simulink model "sparam_filter_rab"  (Simulink 7.4)
settings: Solver=ode45  StartTime=0.0  StopTime=10  RelTol=1e-3
undefined symbols (not defined in the file or in its folder): Fs, magnitude, read, rfdata
libraries: dspindex x6, dspsigops x3, dspsnks4 x2, rfports1 x2, dspbuff3 x2, dspxfrm3 x2, dsparch3 x2, rfblackbox1 x1, simulink x1, dspmtrx3 x1, dspsrcs4 x1
settings Model: Creator=mikem  LastModifiedBy=Dick
settings DataIOCC: SaveOutput=off  SaveTime=off  SignalLoggingName=sigsOut
settings OptimizationCC: InlineInvariantSignals=on  InitFltsAndDblsToZero=on
settings DebuggingCC: SaveWithParameterizedLinksMsg=none  CheckExecutionContextPreStartOutputMsg=on  CheckExecutionContextRuntimeOutputMsg=on  SignalResolutionControl=TryResolveAllWithWarning  SolverPrmCheckMsg=none  MultiTaskDSMMsg=warning  MultiTaskCondExecSysMsg=none  StrictBusMsg=None
settings HardwareCC: ProdHWDeviceType=Specified
settings ModelReferenceCC: UpdateModelReferenceTargets=IfOutOfDate
settings RTWCC: IncludeERTFirstTime=on
settings GRTTargetCC: TargetFcnLib=ansi_tfl_tmw.mat

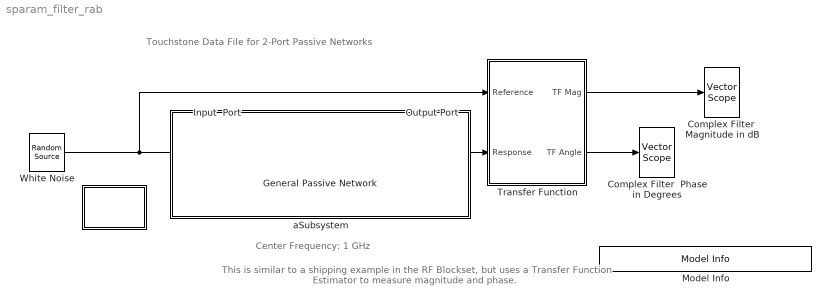
== system sparam_filter_rab ==
  note: Touchstone Data File for 2-Port Passive Networks
  note: Center Frequency: 1 GHz
  note: This is similar to a shipping example in the RF Blockset, but uses a
      | Transfer Function Estimator to measure magnitude and phase.
  " " : Subsystem
      mask Type: Interpolation filter info block
      mask Display: disp('Info')
  Complex Filter  Phase in Degrees : dspsnks4/Vector Scope  DialogController=dspdialog.VectorScope  DialogControllerArgs=DataTag0  ScopeProperties=on  Domain=Frequency  HorizSpan=1  DisplayProperties=off  AxisGrid=on  Memory=off  FrameNumber=on  AxisLegend=off  AxisZoom=off  OpenScopeAtSimStart=on  OpenScopeImmediately=off  FigPos=[403 451 372 236]  AxisProperties=off  XUnits=Hertz  XRange=[-Fs/2...Fs/2]  InheritXIncr=on  XIncr=1  XLabel=Frequency  XLimit=Auto  XMin=0  XMax=1  XStart=0  YUnits=Magnitude  YLabel=Phase in Degrees  LineProperties=off  XAxisParamsVer=6.8
      settings: YMin=3.94458364257076  YMax=51.3691046575291
  Complex Filter  Magnitude in dB : dspsnks4/Vector Scope  DialogController=dspdialog.VectorScope  DialogControllerArgs=DataTag1  ScopeProperties=on  Domain=Frequency  HorizSpan=1  DisplayProperties=off  AxisGrid=on  Memory=off  FrameNumber=on  AxisLegend=off  AxisZoom=off  OpenScopeAtSimStart=on  OpenScopeImmediately=off  FigPos=[22 454 372 232]  AxisProperties=off  XUnits=Hertz  XRange=[-Fs/2...Fs/2]  InheritXIncr=on  XIncr=2*Fs  XLabel=Time  XLimit=Auto  XMin=0  XMax=1  XStart=0  YUnits=dB  YLabel=dB  LineProperties=off  LineColors=[0 0 0]|[1 0 0]  XAxisParamsVer=6.8
      settings: YMin=-30  YMax=-10
  General Passive Network : rfblackbox1/General Passive Network  DialogController=rfblksDDGCreate  DialogControllerArgs=DataTag2  PhysicalDomain=rfsystemsdomain  SubClassName=general-passive-network  LeftPortType=p1  RightPortType=p1  LConnTagsString=__newl0  RConnTagsString=__newr0  DataSource=RFDATA object  RFDATA=read(rfdata.data, 'passive.s2p')  File=passive.s2p  InterpMethod=Linear  PlotFreq=Derived from Input Port parameters  SourceFreq=Extracted from data source  Freq=[0.3e6:0.1e6:6e9]  AllPlotType=Composite data  AppliedNetworkData=S11  AppliedComplexFormat=Magnitude (decibels)  AppliedNetworkData2=""  AppliedXParameter=Freq  AppliedXFormat=Hz  YOption=Linear  XOption=Linear  PlotZ0=50  PlotFreqNoSim=Extracted from RFDATA object  DisplayData=off  NetworkData=S21  SmithData=S11  PolarData=S11  ComplexFormat=Magnitude (decibels)  DBFormat=Magnitude (decibels)  NoneFormat=None
  Input  Port : rfports1/Input Port  Description=source block  DialogController=rfblksDDGCreate  DialogControllerArgs=DataTag3  SystemSampleTime=-1  TreatSimulinkInputSignalAs=Source voltage  MaxLength=160  FracBW=0  ModelDelay=0  Fc=1e9  Ts=0.5e-9  Zs=50  NoiseFlag=off  seed=67987  GoToTag=ACCBGAFQQLCICJWLUPHEIUK
  Model Info : simulink/Model-Wide Utilities/Model Info  SystemSampleTime=-1  InitialBlockCM=None  BlockCM=None  Frame=on  DisplayStringWithTags=Copywrite 2005-2010 The MathWorks, Inc.  HorizontalTextAlignment=Center  LeftAlignmentValue=0.5  SourceBlockDiagram=sparam_filter_rab  TagMaxNumber=20
  Output Port : rfports1/Output Port  DialogController=rfblksDDGCreate  DialogControllerArgs=DataTag4  SystemSampleTime=-1  Zl=50  Flag=1  num_Models=1  GoToTag=ACCBGAFQQLCICJWLUPHEIUK  PlotFreq=Derived from Input Port parameters  SourceFreq=Derived from Input Port parameters  Freq=1e9:1e8:3e9  AllPlotType=Composite data  AppliedNetworkData=S11  AppliedComplexFormat=Magnitude (decibels)  AppliedNetworkData2=""  AppliedXParameter=Freq  AppliedXFormat=Hz  YOption=Linear  XOption=Linear  PlotZ0=50  DisplayData=off  NoBudgetPlot=Composite data  NetworkData=S11  SmithData=S11  PolarData=S11  ComplexFormat=Magnitude (decibels)  DBFormat=Magnitude (decibels)  DBMFormat=dBm  NoneFormat=None
  "Transfer Function " : Subsystem  mask{NFFT=1024, Navg=100, pcnt=100/1.28, unwrap_flag=on}
      mask prompts: NFFT "FFT length (power of 2):"; Navg "Spectral Averaging Factor (>=1):"; pcnt "Percentage of  Alias Free Data  (<=100)"; unwrap_flag "Unwrap Phase"
      mask Display: disp('Transfer Function \n Estimation (v2.0) ')
  White Noise : dspsrcs4/Random Source  SrcType=Gaussian  NormMethod=Ziggurat  CltLength=12  MinVal=-1.25  MaxVal=1.25  MeanVal=0  VarVal=1  RepMode=Not repeatable  rawSeed=1  IsInherit=off  SampMode=Discrete  SampTime=0.5e-9  SampFrame=256  DataType=Double  OutComplex=Complex
  aSubsystem : Subsystem
      mask Display: disp('')
  wires:
  White Noise/1 -> Input  Port/1, "Transfer Function "/1(Reference)
  Output Port/1 -> "Transfer Function "/2(Response)
  "Transfer Function "/1(TF Mag) -> Complex Filter  Magnitude in dB/1
  "Transfer Function "/2(TF Angle) -> Complex Filter  Phase in Degrees/1
  connections:
  Input  Port/RConn1 -- General Passive Network/LConn1
  General Passive Network/RConn1 -- Output Port/LConn1

== system sparam_filter_rab/  ==
  note: Touchstone Data File for 2-Port Passive Networks
      |
      | The Black Box Elements library has blocks to handle
      | S, Y, and Z parameters of the passive networks.
      | The library also has 'General Passive Network' block
      | that can be used for the Touchstone data file.
      |
      | The data file: 'passive.s2p' has
      | the S-parameters of a 2-port passive network
      | over the frequency range 315KHz to 6GHz.
      | The spectrum plot shows frequency ranging from
      | 0Hz to 2GHz centered at 1GHz.
      |
      |
      | If you want to see the frequency response centered at other RF frequency,
      | you need to change the Center frequency parameter in the
      | 'Input Port' block.
      |
      | If you want to change the range of frequency response that is determined by
      | the Sample time parameter specified in the 'Input Port' and 'White Noise' blocks,
      | you need to change the Sample time parameter in both blocks.

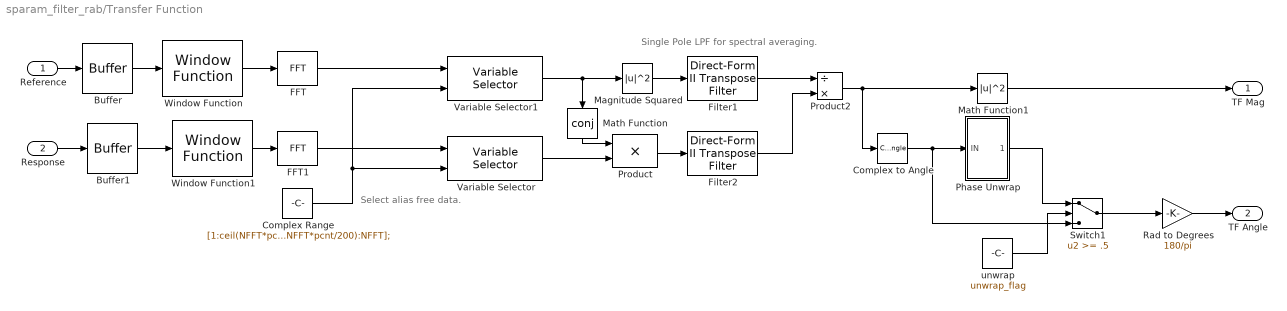
== system sparam_filter_rab/Transfer Function  ==
  note: Single Pole LPF for spectral averaging.
  note: Select alias free data.
  Reference : Inport  OutDataType=sfix(16)  OutScaling=2^0
  Response : Inport  Port=2  OutDataType=sfix(16)  OutScaling=2^0
  Buffer : dspbuff3/Buffer  N=NFFT  V=0  ic=0
  Buffer1 : dspbuff3/Buffer  N=NFFT  V=0  ic=0
  Complex Range : Constant  Value=[1:ceil(NFFT*pcnt/200),ceil(1+NFFT-NFFT*pcnt/200):NFFT];  OutDataType=sfix(16)  OutScaling=2^0
  Complex to Angle : ComplexToMagnitudeAngle  Output=Angle
  FFT : dspxfrm3/FFT  DialogController=dspDDGCreate  DialogControllerArgs=DataTag5  CompMethod=Table lookup  TableOpt=HYBRID  TableOptActive=Speed  BitRevOrder=off  InheritFFTLength=on  FFTLength=64  SkipNorm=on  firstCoeffMode=Specify word length  firstCoeffWordLength=16  firstCoeffFracLength=15  roundingMode=Floor  overflowMode=off
  FFT1 : dspxfrm3/FFT  DialogController=dspDDGCreate  DialogControllerArgs=DataTag6  CompMethod=Table lookup  TableOpt=HYBRID  TableOptActive=Speed  BitRevOrder=off  InheritFFTLength=on  FFTLength=64  SkipNorm=on  firstCoeffMode=User-defined  firstCoeffWordLength=16  firstCoeffFracLength=15  roundingMode=Floor  overflowMode=off
  Filter1 : dsparch3/Direct-Form II Transpose Filter  num=1  den=[Navg -(Navg-1)]  ic=eps
  Filter2 : dsparch3/Direct-Form II Transpose Filter  num=1  den=[Navg -(Navg-1)]  ic=eps
  Magnitude Squared : Math  Operator=magnitude^2  OutDataType=sfix(16)  OutScaling=2^0  SaturateOnIntegerOverflow=on
  Math Function : Math  Operator=conj  OutDataType=sfix(16)  OutScaling=2^0  SaturateOnIntegerOverflow=on
  Math Function1 : Math  Operator=magnitude^2  OutDataType=sfix(16)  OutScaling=2^0  SaturateOnIntegerOverflow=on
  Phase Unwrap : Subsystem
  Product : Product  OutDataType=sfix(16)  OutScaling=2^0  SaturateOnIntegerOverflow=on  InputSameDT=on  OutDataTypeStr=Inherit: Same as first input
  Product2 : Product  Inputs=/*  OutDataType=sfix(16)  OutScaling=2^0  SaturateOnIntegerOverflow=on  InputSameDT=on  OutDataTypeStr=Inherit: Same as first input
  Rad to Degrees : Gain  Gain=180/pi  ParameterDataType=sfix(16)  ParameterScaling=2^0  OutDataType=sfix(16)  OutScaling=2^0
  Switch1 : Switch  Threshold=.5
  Variable Selector : dspindex/Variable Selector  NumInputs=1  rowsOrCols=Rows  IdxMode=Variable  Elements=[1 3]  ZerOneIdxMode=One-based  errmode=Clip Index  FillMode=on  FillValues=0
  Variable Selector1 : dspindex/Variable Selector  NumInputs=1  rowsOrCols=Rows  IdxMode=Variable  Elements=[1 3]  ZerOneIdxMode=One-based  errmode=Clip Index  FillMode=on  FillValues=0
  Window Function : dspsigops/Window Function  DialogController=dspDDGCreate  DialogControllerArgs=DataTag8  winmode=Apply window to input  wintype=Hann  sampmode=Continuous  samptime=1  N=64  Rs=50  beta=10  winsamp=Periodic  UserWindow=hamming  OptParams=off  UserParams={'symmetric'}  dataType=double  isSigned=on  wordLen=16  udDataType=sfix(16)  fracBitsMode=Best precision  numFracBits=15  roundingMode=Floor  overflowMode=off  numSidelobes=4  sidelobeLevel=-30
  Window Function1 : dspsigops/Window Function  DialogController=dspDDGCreate  DialogControllerArgs=DataTag9  winmode=Apply window to input  wintype=Hann  sampmode=Continuous  samptime=1  N=64  Rs=50  beta=10  winsamp=Periodic  UserWindow=hamming  OptParams=off  UserParams={'symmetric'}  dataType=double  isSigned=on  wordLen=16  udDataType=sfix(16)  fracBitsMode=Best precision  numFracBits=15  roundingMode=Floor  overflowMode=off  numSidelobes=4  sidelobeLevel=-30
  unwrap : Constant  Value=unwrap_flag  OutDataType=sfix(16)  OutScaling=2^0
  TF Mag : Outport  OutDataType=sfix(16)  OutScaling=2^0
  TF Angle : Outport  Port=2  OutDataType=sfix(16)  OutScaling=2^0
  wires:
  Complex Range/1 -> Variable Selector/2, Variable Selector1/2
  Complex to Angle/1 -> Switch1/3, Phase Unwrap/1(IN)
  Rad to Degrees/1 -> TF Angle/1
  Response/1 -> Buffer1/1
  Reference/1 -> Buffer/1
  Product/1 -> Filter2/1
  FFT1/1 -> Variable Selector/1
  Math Function/1 -> Product/1
  Magnitude Squared/1 -> Filter1/1
  FFT/1 -> Variable Selector1/1
  Math Function1/1 -> TF Mag/1
  Window Function/1 -> FFT/1
  Window Function1/1 -> FFT1/1
  Filter1/1 -> Product2/1
  Filter2/1 -> Product2/2
  Buffer/1 -> Window Function/1
  Buffer1/1 -> Window Function1/1
  Product2/1 -> Complex to Angle/1, Math Function1/1
  Variable Selector/1 -> Product/2
  Variable Selector1/1 -> Magnitude Squared/1, Math Function/1
  Switch1/1 -> Rad to Degrees/1
  unwrap/1 -> Switch1/2
  Phase Unwrap/1(Out1) -> Switch1/1

== system sparam_filter_rab/aSubsystem ==

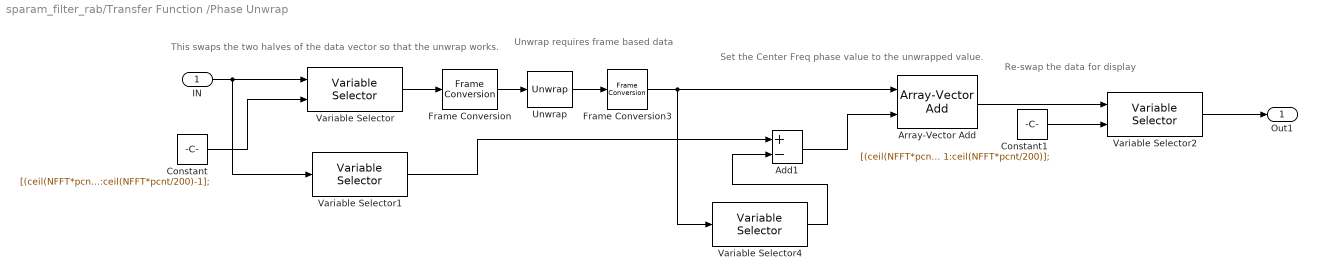
== system sparam_filter_rab/Transfer Function /Phase Unwrap ==
  note: This swaps the two halves of the data vector
      | so that the unwrap works.
  note: Set the Center Freq phase value to the unwrapped value.
  note: Re-swap the data for display
  note: Unwrap requires frame based data
  IN : Inport  OutDataType=sfix(16)  OutScaling=2^0
  Add1 : Sum  Inputs=+-  OutDataType=sfix(16)  OutScaling=2^-10
  Array-Vector Add : dspmtrx3/Array-Vector Add  DialogController=dspDDGCreate  DialogControllerArgs=DataTag7  Dimension=2  V_Source=Input port  V_VectFromMask=[0.5 0.25]  firstCoeffDataTypeStr=Inherit: Same word length as input  firstCoeffLastDataTypeStr=Inherit: Same word length as input  firstCoeffMin=[]  firstCoeffMax=[]  outputDataTypeStr=Inherit: Same as accumulator  outputLastDataTypeStr=Inherit: Same as accumulator  outputMin=[]  outputMax=[]  roundingMode=Floor  overflowMode=off
  Constant : Constant  Value=[(ceil(NFFT*pcnt/200)):ceil(NFFT*pcnt/100) 1:ceil(NFFT*pcnt/200)-1];  OutDataType=sfix(16)  OutScaling=2^0
  Constant1 : Constant  Value=[(ceil(NFFT*pcnt/200)+1):ceil(NFFT*pcnt/100) 1:ceil(NFFT*pcnt/200)];  OutDataType=sfix(16)  OutScaling=2^0
  Frame Conversion : FrameConversion
  Frame Conversion3 : FrameConversion  OutFrame=Sample-based
  Unwrap : dspsigops/Unwrap  running=on  tol=pi
  Variable Selector : dspindex/Variable Selector  NumInputs=1  rowsOrCols=Rows  IdxMode=Variable  Elements=[1 3]  ZerOneIdxMode=One-based  errmode=Clip Index  FillMode=on  FillValues=0
  Variable Selector1 : dspindex/Variable Selector  NumInputs=1  rowsOrCols=Rows  IdxMode=Fixed  Elements=[1]  ZerOneIdxMode=One-based  errmode=Clip Index  FillMode=on  FillValues=0
  Variable Selector2 : dspindex/Variable Selector  NumInputs=1  rowsOrCols=Rows  IdxMode=Variable  Elements=[1 3]  ZerOneIdxMode=One-based  errmode=Clip Index  FillMode=on  FillValues=0
  Variable Selector4 : dspindex/Variable Selector  NumInputs=1  rowsOrCols=Rows  IdxMode=Fixed  Elements=length([(ceil(NFFT*pcnt/200)+1):ceil(NFFT*pcnt/100) 1:ceil(NFFT*pcnt/200)] )/2+1  ZerOneIdxMode=One-based  errmode=Clip Index  FillMode=on  FillValues=0
  Out1 : Outport  OutDataType=sfix(16)  OutScaling=2^0
  wires:
  Frame Conversion/1 -> Unwrap/1
  Variable Selector2/1 -> Out1/1
  IN/1 -> Variable Selector/1, Variable Selector1/1
  Constant/1 -> Variable Selector/2
  Variable Selector/1 -> Frame Conversion/1
  Variable Selector1/1 -> Add1/1
  Unwrap/1 -> Frame Conversion3/1
  Variable Selector4/1 -> Add1/2
  Constant1/1 -> Variable Selector2/2
  Frame Conversion3/1 -> Variable Selector4/1, Array-Vector Add/1
  Add1/1 -> Array-Vector Add/2
  Array-Vector Add/1 -> Variable Selector2/1
